simulink library "css"  (Simulink 8.1)
settings: Solver=ode1  StartTime=0.0  StopTime=Inf  FixedStep=0.001  RelTol=1e-3
PostLoadFcn:
  | , if any(exist('dsrtsu_mdlpostloadfcn', 'file') == [2, 3, 6]), try dsrtsu_mdlpostloadfcn('Execute', bdroot); catch fprintf('Error in PostLoadFcn (dsrtsu_mdlpostloadfcn) for model "%s":\n %s\n', bdroot, lasterr); end, end,
undefined symbols (not defined in the file or in its folder): KJUD_ACCDeactVehSpeed_kph
settings Model: DSRTSU_INTERNAL_RTI_VER=450  DSRTSU_INTERNAL_RTI_TYPE=rti1401  RTICANMMDATA=struct('GeneralSetupData',struct('modelroot','D:\Projects\ELN150201\Repositories\Taiwan\trunk\AdasDragon\software\sw_development\arch\app\jud','generalsettings',struct('filesettings',struct('destfolder',struct('Name','RTICANMM_FILES','Check',1),'buildfolder',struct('Name','.','Check',1),'AbsDestfolder',struct('Name','D:\Projects\ELN150201\Repositories\Taiwan\trunk\AdasDragon\software\sw_development\arch\app\jud\RTICANMM_FILES'),'AbsBuildfolder',struct('Name','D:\Projects\ELN150201\Repositories\Taiwan\trunk\AdasDragon\software\sw_development\arch\app\jud'))),'options',struct('addpaths',1,'rmpaths',1,'addtrcexclusion',logical(1),'cannavigator',struct('checkmonitoring',0),'show_usrtrc',0,'use_usrtrc',0),'advanced',struct('options',[1 1 1 1 1 1 1 1 1 1 1 1 1 1 1 1 1 1 1 1 1 1 1 1 1 1 1 1 1 1 1 1 1 1 1 1 1 1 1 1 1 1 1 1 1 1 1 1 1 1 1 1 1 1 1 1 1 1 1 1 1 1 1 1 1 1 1 1 1 1 1 1 1 1 1 1 1 1 1 1 1 1 1 1 1 1 1 1 1 1 1 1 1 1 1 1 1 1 1 1]),'MPSetup',{{}},'modelname','css','block','css'))  DSRTSU_INTERNAL_RTIFPGA=40  Creator=AT015411  LastModifiedBy=AT015086

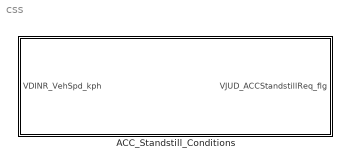
== system css ==
  ACC_Standstill_Conditions : Subsystem

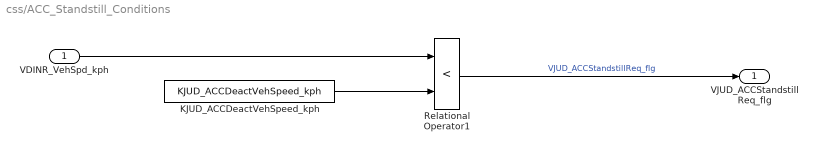
== system css/ACC_Standstill_Conditions ==
  VDINR_VehSpd_kph : Inport
  KJUD_ACCDeactVehSpeed_kph : Constant  Value=KJUD_ACCDeactVehSpeed_kph
  Relational Operator1 : RelationalOperator  Operator=<  OutDataTypeStr=boolean
  VJUD_ACCStandstillReq_flg : Outport
  wires:
  VDINR_VehSpd_kph/1 -> Relational Operator1/1
  Relational Operator1/1 -> VJUD_ACCStandstillReq_flg/1  "VJUD_ACCStandstillReq_flg"
  KJUD_ACCDeactVehSpeed_kph/1 -> Relational Operator1/2
